simulink model "app_Main100msMgr"  (R2016b)
settings: Solver=FixedStepDiscrete  StartTime=0.0  StopTime=10.0  FixedStep=0.001  RelTol=1e-3  EnableMultiTasking=on
PreLoadFcn:
  | try
  |    tapas_types('load');
  | catch
  |   disp('TAPAS WARNING: Tapas Types could not be loaded ...');
  | end
  | 
  | try
  |   app_types('load');
  | catch
  |   currdir =pwd;
  |   try
  |     cd('..\app_types\');
  |     app_types('load');
  |     cd(currdir);
  |   catch
  |     try
  |        cd('..\..\app_types\');
  |        app_types('load');
  |        cd(currdir);
  |     catch
  |        cd(currdir);
  |        disp('TAPAS WARNING: Application Types could not be loaded ...');
  |     end
  |   end
  |   try
  |       clear currdir;
  |   catch
  |      %Do nothing
  |   end
  | end
libraries: Lib_ICAT_VCU_Com x76, Lib_ICAT_VCU_IO x12, simulink x2, Lib_ICAT_VCU_Anlg x1
(part 2 of 2)

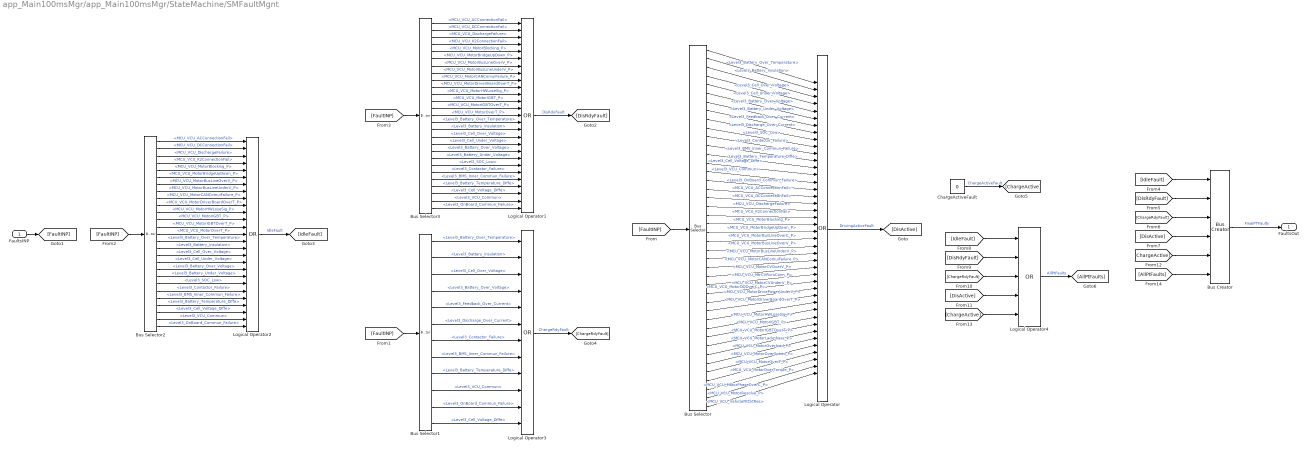
== system app_Main100msMgr/app_Main100msMgr/StateMachine/SMFaultMgnt ==
  FaultsINP : Inport
  Bus Creator : BusCreator  Inputs=6
  Bus Selector : BusSelector  OutputSignals=BMS_Faults.BMS_Level3_Faults.Level3_Battery_Over_Temperature,BMS_Faults.BMS_Level3_Faults.Level3_Battery_Insulation,BMS_Faults.BMS_Level3_Faults.Level3_Cell_Over_Voltage,BMS_Faults.BMS_Level3_Faults.Level3_Cell_Under_Voltage,BMS_Faults.BMS_Level3_Faults.Level3_Battery_Over_Voltage,BMS_Faults.BMS_Level3_Faults.Level3_Battery_Under_Voltage,BMS_Faults.BMS_Level3_Faults.Level3_Feedback_Over_Current,BMS_Faults.BMS_Level3_Faults.Level3_Discharge_Over_Current,BMS_Faults.BMS_Level3_Faults.Level3_SOC_Low,BMS_Faults.BMS_Level3_Faults.Level3_Contactor_Failure,BMS_Faults.BMS_Level3_Faults.Level3_BMS_Inner_Commun_Failure,BMS_Faults.BMS_Level3_Faults.Level3_Battery_Temperature_Diffe,BMS_Faults.BMS_Level3_Faults.Level3_Cell_Voltage_Diffe,BMS_Faults.BMS_Level3_Faults.Level3_VCU_Commun,BMS_Faults.BMS_Level3_Faults.Level3_OnBoard_Commun_Failure,MCU_Faults.MCU_VCU_ACConnectionFail,MCU_Faults.MCU_VCU_DCConnectionFail,MCU_Faults.MCU_VCU_DischargeFailure,MCU_Faults.MCU_VCU_K2ConnectionFail,MCU_Faults.MCU_VCU_MotorBlocking_P,MCU_Faults.MCU_VCU_MotorBridgeUpDown_P,MCU_Faults.MCU_VCU_MotorBusLineOverC_P,MCU_Faults.MCU_VCU_MotorBusLineOverV_P,MCU_Faults.MCU_VCU_MotorBusLineUnderV_P,MCU_Faults.MCU_VCU_MotorCANComuiFailure_P,MCU_Faults.MCU_VCU_MotorCVOverV_P,MCU_Faults.MCU_VCU_MtrCVRvrsConn_P,MCU_Faults.MCU_VCU_MotorCVUnderV_P,MCU_Faults.MCU_VCU_MotorDQOverC_P,MCU_Faults.MCU_VCU_MotorDrivePowerUnderV_P,MCU_Faults.MCU_VCU_MotorDriverBoardOverT_P,MCU_Faults.MCU_VCU_MotorHWLoseSig_P,MCU_Faults.MCU_VCU_MotorIGBT_P,MCU_Faults.MCU_VCU_MotorIGBTOverT_P,MCU_Faults.MCU_VCU_MotorLackphase_P,MCU_Faults.MCU_VCU_MotorOverload_P,MCU_Faults.MCU_VCU_MotorOverSpeed_P,MCU_Faults.MCU_VCU_MotorOverT_P,MCU_Faults.MCU_VCU_MotorOverTorque_P,MCU_Faults.MCU_VCU_MotorPhaseOverC_P,MCU_Faults.MCU_VCU_MotorResolve_P,MCU_Faults.MCU_VCU_VehicleFltCktRes
  Bus Selector1 : BusSelector  OutputSignals=BMS_Faults.BMS_Level3_Faults.Level3_Battery_Over_Temperature,BMS_Faults.BMS_Level3_Faults.Level3_Battery_Insulation,BMS_Faults.BMS_Level3_Faults.Level3_Cell_Over_Voltage,BMS_Faults.BMS_Level3_Faults.Level3_Battery_Over_Voltage,BMS_Faults.BMS_Level3_Faults.Level3_Feedback_Over_Current,BMS_Faults.BMS_Level3_Faults.Level3_Discharge_Over_Current,BMS_Faults.BMS_Level3_Faults.Level3_Contactor_Failure,BMS_Faults.BMS_Level3_Faults.Level3_BMS_Inner_Commun_Failure,BMS_Faults.BMS_Level3_Faults.Level3_Battery_Temperature_Diffe,BMS_Faults.BMS_Level3_Faults.Level3_VCU_Commun,BMS_Faults.BMS_Level3_Faults.Level3_OnBoard_Commun_Failure,BMS_Faults.BMS_Level3_Faults.Level3_Cell_Voltage_Diffe
  Bus Selector2 : BusSelector  OutputSignals=MCU_Faults.MCU_VCU_ACConnectionFail,MCU_Faults.MCU_VCU_DCConnectionFail,MCU_Faults.MCU_VCU_DischargeFailure,MCU_Faults.MCU_VCU_K2ConnectionFail,MCU_Faults.MCU_VCU_MotorBlocking_P,MCU_Faults.MCU_VCU_MotorBridgeUpDown_P,MCU_Faults.MCU_VCU_MotorBusLineOverV_P,MCU_Faults.MCU_VCU_MotorBusLineUnderV_P,MCU_Faults.MCU_VCU_MotorCANComuiFailure_P,MCU_Faults.MCU_VCU_MotorDriverBoardOverT_P,MCU_Faults.MCU_VCU_MotorHWLoseSig_P,MCU_Faults.MCU_VCU_MotorIGBT_P,MCU_Faults.MCU_VCU_MotorIGBTOverT_P,MCU_Faults.MCU_VCU_MotorOverT_P,BMS_Faults.BMS_Level3_Faults.Level3_Battery_Over_Temperature,BMS_Faults.BMS_Level3_Faults.Level3_Battery_Insulation,BMS_Faults.BMS_Level3_Faults.Level3_Cell_Over_Voltage,BMS_Faults.BMS_Level3_Faults.Level3_Cell_Under_Voltage,BMS_Faults.BMS_Level3_Faults.Level3_Battery_Over_Voltage,BMS_Faults.BMS_Level3_Faults.Level3_Battery_Under_Voltage,BMS_Faults.BMS_Level3_Faults.Level3_SOC_Low,BMS_Faults.BMS_Level3_Faults.Level3_Contactor_Failure,BMS_Faults.BMS_Level3_Faults.Level3_BMS_Inner_Commun_Failure,BMS_Faults.BMS_Level3_Faults.Level3_Battery_Temperature_Diffe,BMS_Faults.BMS_Level3_Faults.Level3_Cell_Voltage_Diffe,BMS_Faults.BMS_Level3_Faults.Level3_VCU_Commun,BMS_Faults.BMS_Level3_Faults.Level3_OnBoard_Commun_Failure
  Bus Selector3 : BusSelector  OutputSignals=MCU_Faults.MCU_VCU_ACConnectionFail,MCU_Faults.MCU_VCU_DCConnectionFail,MCU_Faults.MCU_VCU_DischargeFailure,MCU_Faults.MCU_VCU_K2ConnectionFail,MCU_Faults.MCU_VCU_MotorBlocking_P,MCU_Faults.MCU_VCU_MotorBridgeUpDown_P,MCU_Faults.MCU_VCU_MotorBusLineOverV_P,MCU_Faults.MCU_VCU_MotorBusLineUnderV_P,MCU_Faults.MCU_VCU_MotorCANComuiFailure_P,MCU_Faults.MCU_VCU_MotorDriverBoardOverT_P,MCU_Faults.MCU_VCU_MotorHWLoseSig_P,MCU_Faults.MCU_VCU_MotorIGBT_P,MCU_Faults.MCU_VCU_MotorIGBTOverT_P,MCU_Faults.MCU_VCU_MotorOverT_P,BMS_Faults.BMS_Level3_Faults.Level3_Battery_Over_Temperature,BMS_Faults.BMS_Level3_Faults.Level3_Battery_Insulation,BMS_Faults.BMS_Level3_Faults.Level3_Cell_Over_Voltage,BMS_Faults.BMS_Level3_Faults.Level3_Cell_Under_Voltage,BMS_Faults.BMS_Level3_Faults.Level3_Battery_Over_Voltage,BMS_Faults.BMS_Level3_Faults.Level3_Battery_Under_Voltage,BMS_Faults.BMS_Level3_Faults.Level3_SOC_Low,BMS_Faults.BMS_Level3_Faults.Level3_Contactor_Failure,BMS_Faults.BMS_Level3_Faults.Level3_BMS_Inner_Commun_Failure,BMS_Faults.BMS_Level3_Faults.Level3_Battery_Temperature_Diffe,BMS_Faults.BMS_Level3_Faults.Level3_Cell_Voltage_Diffe,BMS_Faults.BMS_Level3_Faults.Level3_VCU_Commun,BMS_Faults.BMS_Level3_Faults.Level3_OnBoard_Commun_Failure
  ChargeActiveFault : Constant  Value=0
  Logical Operator : Logic  Operator=OR  Inputs=42  AllPortsSameDT=off  OutDataTypeStr=boolean
  Logical Operator1 : Logic  Operator=OR  Inputs=27  AllPortsSameDT=off  OutDataTypeStr=boolean
  Logical Operator2 : Logic  Operator=OR  Inputs=27  AllPortsSameDT=off  OutDataTypeStr=boolean
  Logical Operator3 : Logic  Operator=OR  Inputs=12  AllPortsSameDT=off  OutDataTypeStr=boolean
  Logical Operator4 : Logic  Operator=OR  Inputs=5  AllPortsSameDT=off  OutDataTypeStr=boolean
  FaultsOut : Outport
  wires:
  Logical Operator/1 -> [DisActive]  "DrivingActiveFault"
  Bus Selector/1 -> Logical Operator/1  "<Level3_Battery_Over_Temperature>"
  Bus Selector/2 -> Logical Operator/2  "<Level3_Battery_Insulation>"
  Bus Selector/3 -> Logical Operator/3  "<Level3_Cell_Over_Voltage>"
  Bus Selector/4 -> Logical Operator/4  "<Level3_Cell_Under_Voltage>"
  Bus Selector/5 -> Logical Operator/5  "<Level3_Battery_Over_Voltage>"
  Bus Selector/6 -> Logical Operator/6  "<Level3_Battery_Under_Voltage>"
  Bus Selector/7 -> Logical Operator/7  "<Level3_Feedback_Over_Current>"
  Bus Selector/8 -> Logical Operator/8  "<Level3_Discharge_Over_Current>"
  Bus Selector/9 -> Logical Operator/9  "<Level3_SOC_Low>"
  Bus Selector/10 -> Logical Operator/10  "<Level3_Contactor_Failure>"
  Bus Selector/11 -> Logical Operator/11  "<Level3_BMS_Inner_Commun_Failure>"
  Bus Selector/12 -> Logical Operator/12  "<Level3_Battery_Temperature_Diffe>"
  Bus Selector/13 -> Logical Operator/13  "<Level3_Cell_Voltage_Diffe>"
  Bus Selector/14 -> Logical Operator/14  "<Level3_VCU_Commun>"
  Bus Selector/15 -> Logical Operator/15  "<Level3_OnBoard_Commun_Failure>"
  Bus Selector/16 -> Logical Operator/16  "<MCU_VCU_ACConnectionFail>"
  Bus Selector/17 -> Logical Operator/17  "<MCU_VCU_DCConnectionFail>"
  Bus Selector/18 -> Logical Operator/18  "<MCU_VCU_DischargeFailure>"
  Bus Selector/19 -> Logical Operator/19  "<MCU_VCU_K2ConnectionFail>"
  Bus Selector/20 -> Logical Operator/20  "<MCU_VCU_MotorBlocking_P>"
  Bus Selector/21 -> Logical Operator/21  "<MCU_VCU_MotorBridgeUpDown_P>"
  Bus Selector/22 -> Logical Operator/22  "<MCU_VCU_MotorBusLineOverC_P>"
  Bus Selector/23 -> Logical Operator/23  "<MCU_VCU_MotorBusLineOverV_P>"
  Bus Selector/24 -> Logical Operator/24  "<MCU_VCU_MotorBusLineUnderV_P>"
  Bus Selector/25 -> Logical Operator/25  "<MCU_VCU_MotorCANComuiFailure_P>"
  Bus Selector/26 -> Logical Operator/26  "<MCU_VCU_MotorCVOverV_P>"
  Bus Selector/27 -> Logical Operator/27  "<MCU_VCU_MtrCVRvrsConn_P>"
  Bus Selector/28 -> Logical Operator/28  "<MCU_VCU_MotorCVUnderV_P>"
  Bus Selector/29 -> Logical Operator/29  "<MCU_VCU_MotorDQOverC_P>"
  Bus Selector/30 -> Logical Operator/30  "<MCU_VCU_MotorDrivePowerUnderV_P>"
  Bus Selector/31 -> Logical Operator/31  "<MCU_VCU_MotorDriverBoardOverT_P>"
  Bus Selector/32 -> Logical Operator/32  "<MCU_VCU_MotorHWLoseSig_P>"
  Bus Selector/33 -> Logical Operator/33  "<MCU_VCU_MotorIGBT_P>"
  Bus Selector/34 -> Logical Operator/34  "<MCU_VCU_MotorIGBTOverT_P>"
  Bus Selector/35 -> Logical Operator/35  "<MCU_VCU_MotorLackphase_P>"
  Bus Selector/36 -> Logical Operator/36  "<MCU_VCU_MotorOverload_P>"
  Bus Selector/37 -> Logical Operator/37  "<MCU_VCU_MotorOverSpeed_P>"
  Bus Selector/38 -> Logical Operator/38  "<MCU_VCU_MotorOverT_P>"
  Bus Selector/39 -> Logical Operator/39  "<MCU_VCU_MotorOverTorque_P>"
  Bus Selector/40 -> Logical Operator/40  "<MCU_VCU_MotorPhaseOverC_P>"
  Bus Selector/41 -> Logical Operator/41  "<MCU_VCU_MotorResolve_P>"
  Bus Selector/42 -> Logical Operator/42  "<MCU_VCU_VehicleFltCktRes>"
  FaultsINP/1 -> [FaultINP]
  [FaultINP] -> Bus Selector/1
  [FaultINP] -> Bus Selector2/1
  Bus Selector2/1 -> Logical Operator2/1  "<MCU_VCU_ACConnectionFail>"
  Bus Selector2/2 -> Logical Operator2/2  "<MCU_VCU_DCConnectionFail>"
  Bus Selector2/3 -> Logical Operator2/3  "<MCU_VCU_DischargeFailure>"
  Bus Selector2/4 -> Logical Operator2/4  "<MCU_VCU_K2ConnectionFail>"
  Bus Selector2/5 -> Logical Operator2/5  "<MCU_VCU_MotorBlocking_P>"
  Bus Selector2/6 -> Logical Operator2/6  "<MCU_VCU_MotorBridgeUpDown_P>"
  Bus Selector2/7 -> Logical Operator2/7  "<MCU_VCU_MotorBusLineOverV_P>"
  Bus Selector2/8 -> Logical Operator2/8  "<MCU_VCU_MotorBusLineUnderV_P>"
  Bus Selector2/9 -> Logical Operator2/9  "<MCU_VCU_MotorCANComuiFailure_P>"
  Bus Selector2/10 -> Logical Operator2/10  "<MCU_VCU_MotorDriverBoardOverT_P>"
  Bus Selector2/11 -> Logical Operator2/11  "<MCU_VCU_MotorHWLoseSig_P>"
  Bus Selector2/12 -> Logical Operator2/12  "<MCU_VCU_MotorIGBT_P>"
  Bus Selector2/13 -> Logical Operator2/13  "<MCU_VCU_MotorIGBTOverT_P>"
  Bus Selector2/14 -> Logical Operator2/14  "<MCU_VCU_MotorOverT_P>"
  Bus Selector2/15 -> Logical Operator2/15  "<Level3_Battery_Over_Temperature>"
  Bus Selector2/16 -> Logical Operator2/16  "<Level3_Battery_Insulation>"
  Bus Selector2/17 -> Logical Operator2/17  "<Level3_Cell_Over_Voltage>"
  Bus Selector2/18 -> Logical Operator2/18  "<Level3_Cell_Under_Voltage>"
  Bus Selector2/19 -> Logical Operator2/19  "<Level3_Battery_Over_Voltage>"
  Bus Selector2/20 -> Logical Operator2/20  "<Level3_Battery_Under_Voltage>"
  Bus Selector2/21 -> Logical Operator2/21  "<Level3_SOC_Low>"
  Bus Selector2/22 -> Logical Operator2/22  "<Level3_Contactor_Failure>"
  Bus Selector2/23 -> Logical Operator2/23  "<Level3_BMS_Inner_Commun_Failure>"
  Bus Selector2/24 -> Logical Operator2/24  "<Level3_Battery_Temperature_Diffe>"
  Bus Selector2/25 -> Logical Operator2/25  "<Level3_Cell_Voltage_Diffe>"
  Bus Selector2/26 -> Logical Operator2/26  "<Level3_VCU_Commun>"
  Bus Selector2/27 -> Logical Operator2/27  "<Level3_OnBoard_Commun_Failure>"
  Logical Operator1/1 -> [DisRdyFault]  "DisRdyFault"
  Logical Operator2/1 -> [IdleFault]  "IdleFault"
  Bus Selector3/27 -> Logical Operator1/27  "<Level3_OnBoard_Commun_Failure>"
  Bus Selector3/26 -> Logical Operator1/26  "<Level3_VCU_Commun>"
  Bus Selector3/25 -> Logical Operator1/25  "<Level3_Cell_Voltage_Diffe>"
  Bus Selector3/24 -> Logical Operator1/24  "<Level3_Battery_Temperature_Diffe>"
  Bus Selector3/23 -> Logical Operator1/23  "<Level3_BMS_Inner_Commun_Failure>"
  Bus Selector3/22 -> Logical Operator1/22  "<Level3_Contactor_Failure>"
  Bus Selector3/21 -> Logical Operator1/21  "<Level3_SOC_Low>"
  Bus Selector3/20 -> Logical Operator1/20  "<Level3_Battery_Under_Voltage>"
  Bus Selector3/19 -> Logical Operator1/19  "<Level3_Battery_Over_Voltage>"
  Bus Selector3/18 -> Logical Operator1/18  "<Level3_Cell_Under_Voltage>"
  Bus Selector3/17 -> Logical Operator1/17  "<Level3_Cell_Over_Voltage>"
  Bus Selector3/16 -> Logical Operator1/16  "<Level3_Battery_Insulation>"
  Bus Selector3/15 -> Logical Operator1/15  "<Level3_Battery_Over_Temperature>"
  Bus Selector3/14 -> Logical Operator1/14  "<MCU_VCU_MotorOverT_P>"
  Bus Selector3/13 -> Logical Operator1/13  "<MCU_VCU_MotorIGBTOverT_P>"
  Bus Selector3/12 -> Logical Operator1/12  "<MCU_VCU_MotorIGBT_P>"
  Bus Selector3/11 -> Logical Operator1/11  "<MCU_VCU_MotorHWLoseSig_P>"
  Bus Selector3/10 -> Logical Operator1/10  "<MCU_VCU_MotorDriverBoardOverT_P>"
  Bus Selector3/9 -> Logical Operator1/9  "<MCU_VCU_MotorCANComuiFailure_P>"
  Bus Selector3/8 -> Logical Operator1/8  "<MCU_VCU_MotorBusLineUnderV_P>"
  Bus Selector3/7 -> Logical Operator1/7  "<MCU_VCU_MotorBusLineOverV_P>"
  Bus Selector3/6 -> Logical Operator1/6  "<MCU_VCU_MotorBridgeUpDown_P>"
  Bus Selector3/5 -> Logical Operator1/5  "<MCU_VCU_MotorBlocking_P>"
  Bus Selector3/4 -> Logical Operator1/4  "<MCU_VCU_K2ConnectionFail>"
  Bus Selector3/3 -> Logical Operator1/3  "<MCU_VCU_DischargeFailure>"
  Bus Selector3/2 -> Logical Operator1/2  "<MCU_VCU_DCConnectionFail>"
  Bus Selector3/1 -> Logical Operator1/1  "<MCU_VCU_ACConnectionFail>"
  [FaultINP] -> Bus Selector3/1
  [FaultINP] -> Bus Selector1/1
  Bus Selector1/1 -> Logical Operator3/1  "<Level3_Battery_Over_Temperature>"
  Bus Selector1/2 -> Logical Operator3/2  "<Level3_Battery_Insulation>"
  Bus Selector1/3 -> Logical Operator3/3  "<Level3_Cell_Over_Voltage>"
  Bus Selector1/4 -> Logical Operator3/4  "<Level3_Battery_Over_Voltage>"
  Bus Selector1/5 -> Logical Operator3/5  "<Level3_Feedback_Over_Current>"
  Bus Selector1/6 -> Logical Operator3/6  "<Level3_Discharge_Over_Current>"
  Bus Selector1/7 -> Logical Operator3/7  "<Level3_Contactor_Failure>"
  Bus Selector1/8 -> Logical Operator3/8  "<Level3_BMS_Inner_Commun_Failure>"
  Bus Selector1/9 -> Logical Operator3/9  "<Level3_Battery_Temperature_Diffe>"
  Bus Selector1/10 -> Logical Operator3/10  "<Level3_VCU_Commun>"
  Bus Selector1/11 -> Logical Operator3/11  "<Level3_OnBoard_Commun_Failure>"
  Bus Selector1/12 -> Logical Operator3/12  "<Level3_Cell_Voltage_Diffe>"
  Logical Operator3/1 -> [ChargeRdyFault]  "ChargeRdyFault"
  [IdleFault] -> Bus Creator/1
  [DisRdyFault] -> Bus Creator/2
  [ChargeRdyFault] -> Bus Creator/3
  [DisActive] -> Bus Creator/4
  Bus Creator/1 -> FaultsOut/1  "FinalPTFaults"
  [IdleFault] -> Logical Operator4/1
  [DisRdyFault] -> Logical Operator4/2
  [ChargeRdyFault] -> Logical Operator4/3
  [DisActive] -> Logical Operator4/4
  ChargeActiveFault/1 -> [ChargeActive]  "ChargeActiveFault"
  [ChargeActive] -> Bus Creator/5
  [ChargeActive] -> Logical Operator4/5
  Logical Operator4/1 -> [AllPtFaults]  "AllPtFaults"
  [AllPtFaults] -> Bus Creator/6

== stateflow chart app_Main100msMgr/MCUAUXRelayManager/PDU_4in1_Handler/Chart ==
  state OFF
    en, du: PrechargeK6 = 0;
    MainPosK7 = 0;
    MainNegK7 = 0;
    MainPosK5 = 0;
    MainPosK4 = 0;
  state NEGK7ON
    en, du:PrechargeK6 = 1;
    MainPosK7 = 1;
    MainNegK7 = 1;
    MainPosK4 = 1;
    MainPosK5 = 0;
  state PosK7ON
    en, du:PrechargeK6 = 0;
    MainPosK7 = 1;
    MainNegK7 = 1;
    MainPosK5 = 1;
    MainPosK4 = 1;
  (default) -> OFF
  (junction 21) -> OFF
  (junction 18) -> (junction 21)
  OFF -> NEGK7ON : [KeyPos == 1 || KeyPos == 2]
  NEGK7ON -> (junction 18) [order 2] : [KeyPos ~= 1 && KeyPos ~= 2]
  (junction 16) -> (junction 18)
  NEGK7ON -> PosK7ON [order 1] : after(3, sec)
  PosK7ON -> (junction 16) [order 1] : [KeyPos ~= 1 && KeyPos ~= 2]
  PosK7ON -> PosK7ON [order 2] : [KeyPos == 1 || KeyPos == 2]
  data: KeyPos input; MainPosK7 output; MainPosK5 output; MainNegK7 output; PrechargeK6 output; MainPosK4 output

== stateflow chart app_Main100msMgr/GearManager/Gear ==
  state Backward
    du : GER_GearState = -1;
  state Forward
    du : GER_GearState = 1;
  (default) -> Forward
  Forward -> Backward : [Di_Gear_RW && Stopped]
  Backward -> Forward : [Di_Gear_FW && Stopped]
  data: Di_Gear_FW input; Di_Gear_RW input; Stopped input; GER_GearState output

== stateflow chart app_Main100msMgr/APP_manager/PedalCondtionChecking2 ==
  state PedalOK
    du:short2ground=0;
    du:short2Vcc=0;
    du:PedalFault=0;
  state PedalFault
    entry: PedalFault=1;
    state short2ground
      du:short2ground=1;
      du:short2Vcc=0;
    state short2Vcc
      du:short2ground=0;
      du:short2Vcc=1;
  (default) -> PedalOK
  (junction 26) -> PedalOK : [voltage > Shor2GndVoltage]
  PedalOK -> short2ground [order 1] : [voltage < Shor2GndVoltage]
  (junction 28) -> PedalOK : [voltage < Shor2VccVoltage]
  PedalOK -> short2Vcc [order 2] : [voltage > Shor2VccVoltage]
  short2ground -> (junction 26) : [CLR_short2ground]
  short2Vcc -> (junction 28) : [CLR_Short2Vcc]
  data: Shor2VccVoltage input; Shor2GndVoltage input; voltage input; short2ground output; short2Vcc output; PedalFault output; CLR_Short2Vcc input; CLR_short2ground input

== stateflow chart app_Main100msMgr/StartKeyMgr/Chart ==
  state Off%No Key Inserted
    entry:
    Key_Position = 0;
  state ACC_ON %key in On position
    entry:  Key_Position = 1;
  state Allow2drive %Temporary in Start position
    state Key3
      entry: Key_Position = 1;
    state Key2
      entry: Key_Position = 2;
    (default) -> Key2
    Key3 -> Key2 : [KeyIn1 && KeyIn2]
    Key2 -> Key3 : [KeyIn1 && ~KeyIn2]
  (default) -> Off%No Key Inserted
  (junction 8) -> Off%No Key Inserted : %delay due to possible zero
      | %crossing between contacts On->Start
      | after(100,msec)
  (junction 22) -> (junction 8) : %if key in not in any detected position
      | [~KeyIn1 && ~KeyIn2]
  (junction 17) -> (junction 22)
  Off%No Key Inserted -> ACC_ON %key in On position : [KeyIn1 == 1]
  ACC_ON %key in On position -> (junction 17) [order 1]
  (junction 11) -> (junction 17)
  ACC_ON %key in On position -> Allow2drive %Temporary in Start position [order 2] : [KeyIn1 && KeyIn2 ]
  Allow2drive %Temporary in Start position -> (junction 11)
  data: KeyIn1 input; KeyIn2 input; Key_Position output

== matlab function app_Main100msMgr/FaultManager/MATLAB Function ==
  data: INP_DEC input; OUT_BIN output
function OUT_BIN = fcn(INP_DEC)
i=1;
a=zeros(1,8);

while INP_DEC >= 2
    r=rem(INP_DEC,2)
    if r==1
        a(i)=1;
    else
        a(i)=0;
    end
    i=i+1;
    INP_DEC=floor(INP_DEC/2);
end
if INP_DEC == 0
    a(i) = 0;
else
    a(i) = 1;
end
OUT_BIN=[a(8),a(7),a(6),a(5),a(4),a(3),a(2),a(1)];

== matlab function app_Main100msMgr/FaultManager/MATLAB Function1 ==
  data: INP_DEC input; OUT_BIN output
function OUT_BIN = fcn(INP_DEC)
i=1;
a=zeros(1,8);

while INP_DEC >= 2
    r=rem(INP_DEC,2)
    if r==1
        a(i)=1;
    else
        a(i)=0;
    end
    i=i+1;
    INP_DEC=floor(INP_DEC/2);
end
if INP_DEC == 0
    a(i) = 0;
else
    a(i) = 1;
end
OUT_BIN=[a(8),a(7),a(6),a(5),a(4),a(3),a(2),a(1)];

== stateflow chart app_Main100msMgr/StateMachine/Chart ==
  state Idle
    en, du: VehicleState = 1;
    DriveActive = 0;
    ChargeActive = 0;
    FaultActive = 0;
    MCUInvCmd = 0;
    state Acc1
      en, du: AccActive = 0;
      MCUVehStatus = 16;
    state Acc
      en, du: AccActive = 1;
      MCUVehStatus = 32;
    (default) -> Acc1
    Acc1 -> Acc : [KeyPos == 1 && ...
        |  AccRdyFault == 0]
    Acc -> Acc1 [order 2] : [KeyPos ~= 1 && ...
        | KeyPos ~= 2]
  state Charging
    en, du: VehicleState = 3;
    DriveActive = 0;
    ChargeActive = 1;
    FaultActive = 0;
    AccActive = 1;
    MCUVehStatus = 80;
  state Driving
    en, du: VehicleState = 2;
    DriveActive = 1;
    ChargeActive = 0;
    FaultActive = 0;
    AccActive = 1;
    MCUVehStatus = 96;
    state VehStop_DriveActive
      en, du: DriveStatus = 0;
      MCUInvCmd = 0;
    state Brakes_Active
      en, du: DriveStatus = 3;
      MCUInvCmd = 0;
    state Coasting_DriveActive
      en, du: DriveStatus = 2;
      MCUInvCmd = 3;
    state Accel_Active
      en, du: DriveStatus = 1;
      MCUInvCmd = 1;
    (default) -> VehStop_DriveActive
    Brakes_Active -> VehStop_DriveActive [order 1] : [MotorRPM ==0 ]
    (junction 61) -> VehStop_DriveActive
    (junction 51) -> Brakes_Active
    (junction 59) -> (junction 61)
    (junction 49) -> (junction 51)
    Brakes_Active -> Coasting_DriveActive [order 2] : [FootBrake ==0 &&...
        |  HndBrake == 0]
    Coasting_DriveActive -> Brakes_Active [order 2] : [FootBrake ~=0 ...
        |  || HndBrake ~= 0]
    VehStop_DriveActive -> Accel_Active : [(APP > 3 && APP <= 100) && ...
        | (FootBrake ==0 && HndBrake == 0)]
    Accel_Active -> Coasting_DriveActive [order 1] : [APP  >=0 && ...
        |  APP <= 3]
    Coasting_DriveActive -> Accel_Active [order 1] : [APP > 3 && ...
        | APP <= 100]
    Accel_Active -> (junction 47) [order 2] : [(FootBrake ~=0 || HndBrake ~= 0) && ...
        | (APP > 3 && APP <= 100) ]
    Coasting_DriveActive -> (junction 57) [order 3] : [MotorRPM == 0]
    (junction 47) -> (junction 49)
    (junction 57) -> (junction 59)
  state Fault
    en, du: VehicleState = 4;
    DriveActive = 0;
    ChargeActive = 0;
    FaultActive = 1;
    AccActive = 1;
    MCUInvCmd = 0;
  (default) -> Idle
  (junction 6) -> Idle
  Idle -> Charging [order 2] : [KeyPos == 0 && HndBrake == 1 && ...
      |  ChargeRdyFault == 0 && ProxCharge == 1]
  (junction 16) -> (junction 6)
  Charging -> Idle [order 2] : [KeyPos ~= 0 || HndBrake ~= 0 || ...
      | ChargedCmpt == 1 || ProxCharge ~= 0 ]
  Idle -> (junction 1) [order 1] : [IdleFault == 1]
  Charging -> Fault [order 1] : [ChargeActiveFault == 1]
  (junction 1) -> (junction 13)
  Acc -> Driving [order 1] : [KeyPos == 2 && ...
      |  DisRdyFault == 0]
  Driving -> Idle [order 2] : [KeyPos <= 1]
  Driving -> Fault [order 1] : [DisActiveFault == 1]
  (junction 7) -> Fault
  Fault -> (junction 12) : [AllFaults == 0]
  (junction 13) -> (junction 7)
  (junction 12) -> (junction 16)
  data: HndBrake input; KeyPos input; AccRdyFault input; DisRdyFault input; ChargeRdyFault input; ProxCharge input; DisActiveFault input; AllFaults input; FootBrake input; ChargedCmpt input; IdleFault input; ChargeActiveFault input; VehicleState output; ChargeActive output; DriveActive output; FaultActive output; AccActive output; APP input; DriveStatus output; MotorRPM input; MCUVehStatus output double; MCUInvCmd output
